simulink model "zajecia3"  (R2022b)
settings: Solver=VariableStepAuto  StartTime=0.0  StopTime=czas_symulacji  RelTol=1e-3
values from neighbouring files (symbols this model uses):
  du = 10    [untitled.m]    (also in zaj3.m = 1)
  t0 = 10    [untitled.m]    (also in zaj3.m)
  u0 = 10    [untitled.m]    (also in zaj3.m = 0)
settings Model: Creator=huber  LastModifiedBy=huber

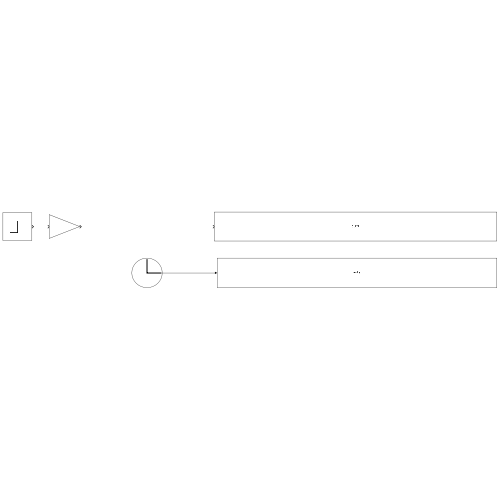
[thumbnail: Simulink's stored preview of the top-level diagram]
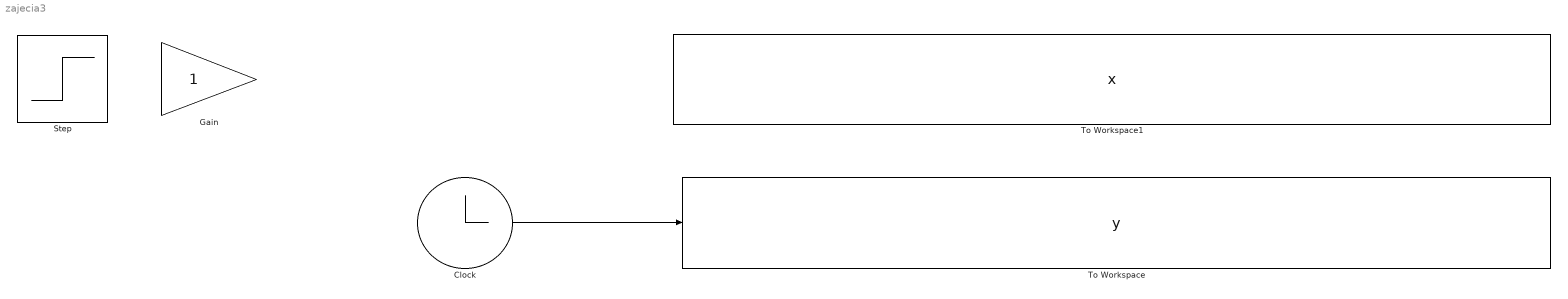
== system zajecia3 ==
  Clock : Clock
  Gain : Gain
  Step : Step  Time=t0  Before=u0  After=du + u0  SampleTime=0
  To Workspace : ToWorkspace  VariableName=y  SampleTime=-1
  To Workspace1 : ToWorkspace  VariableName=x  SampleTime=-1
  wires:
  Clock/1 -> To Workspace/1
